simulink model "ControllerTestModel"  (R2016a)
settings: Solver=FixedStepAuto  StartTime=0.0  StopTime=30  FixedStep=0.01  RelTol=1e-3
settings Model: Creator=Priscilla  LastModifiedBy=Priscilla

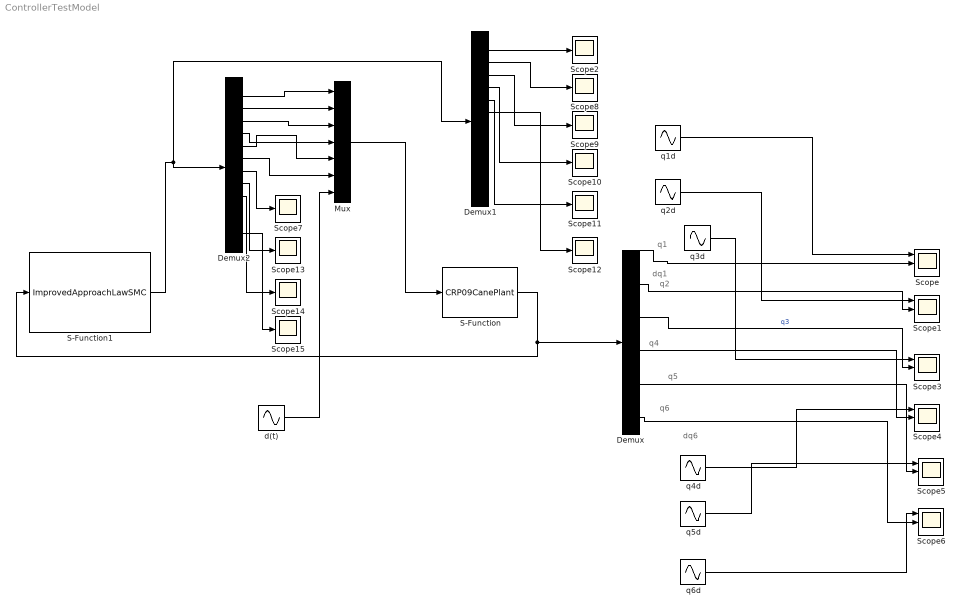
== system ControllerTestModel ==
  note: dq6
  note: q6
  note: q5
  note: q4
  note: q2
  note: dq1
  note: q1
  Demux : Demux  Outputs=12
  Demux1 : Demux  Outputs=12
  Demux2 : Demux  Outputs=12
  Mux : Mux  Inputs=7
  S-Function : S-Function  FunctionName=CRP09CanePlant  SFunctionDeploymentMode=off  EnableBusSupport=off
  S-Function1 : S-Function  FunctionName=ImprovedApproachLawSMC  SFunctionDeploymentMode=off  EnableBusSupport=off
  Scope{,1,3..6} (6 alike) : Scope  NumInputPorts=3
  Scope{2,7..15} (10 alike) : Scope
  d(t) : Sin  Amplitude=10  Frequency=50  SampleTime=0
  q1d : Sin  Frequency=0.25  SampleTime=0
  q2d : Sin  Frequency=0.25  SampleTime=0
  q3d : Sin  Frequency=0.25  SampleTime=0
  q4d : Sin  SampleTime=0
  q5d : Sin  SampleTime=0
  q6d : Sin  SampleTime=0
  wires:
  Demux/1 -> Scope/2
  Demux/3 -> Scope1/2
  Demux/5 -> Scope3/2  "q3"
  Demux/7 -> Scope4/2
  Demux/9 -> Scope5/2
  Demux/11 -> Scope6/2
  Demux2/1 -> Mux/1
  Demux2/2 -> Mux/2
  Demux2/3 -> Mux/3
  Demux2/4 -> Mux/4
  Demux2/5 -> Mux/5
  Demux2/6 -> Mux/6
  S-Function1/1 -> Demux1/1, Demux2/1
  Demux1/1 -> Scope2/1
  Demux1/2 -> Scope8/1
  Demux1/3 -> Scope9/1
  Demux1/4 -> Scope10/1
  Demux1/5 -> Scope11/1
  Demux1/6 -> Scope12/1
  q1d/1 -> Scope/1
  q2d/1 -> Scope1/1
  q3d/1 -> Scope3/1
  q4d/1 -> Scope4/1
  q5d/1 -> Scope5/1
  q6d/1 -> Scope6/1
  d(t)/1 -> Mux/7
  S-Function/1 -> Demux/1, S-Function1/1
  Mux/1 -> S-Function/1
  Demux2/7 -> Scope7/1
  Demux2/8 -> Scope13/1
  Demux2/9 -> Scope14/1
  Demux2/12 -> Scope15/1
